simulink model "PS_03_sim"  (R2018a)
settings: Solver=FixedStepDiscrete  StartTime=0.0  StopTime=2376922056.5209  FixedStep=95076882.2608359  RelTol=1e-3
values from neighbouring files (symbols this model uses):
  a = rp/(1-e)    [AA279A_final2019.m]    (also in ECI2OE.m = inf; OEtoRVv2.m = (mu/n^2)^(1/3); PS_03.m = 2667966400; ps_2.m = sqrt( (L^2-2*T*Ix) / ((Iy-Ix)*Iy) ))
  e = 0.2    [AA279A_final2019.m]    (also in ECI2OE.m = norm ( eVec ); PS_03.m = 0.967; plotParabola.m = 1; ps_2.m = sqrt(1 + (b^2/abs(a^2))))
  M0 = 0    [PS_03.m]
  n = 2*pi/T    [AA279A_final2019.m]    (also in ECI2OE.m = norm ( nVec ); OEtoRV.m = sqrt(mu/a^3); PS_03.m = sqrt(mu/a^3); UDFactor.m = length(P))
  tol = 1E-10    (= 1e-10)    [PS_03.m]
settings Model: Creator=kaitl  LastModifiedBy=kaitl

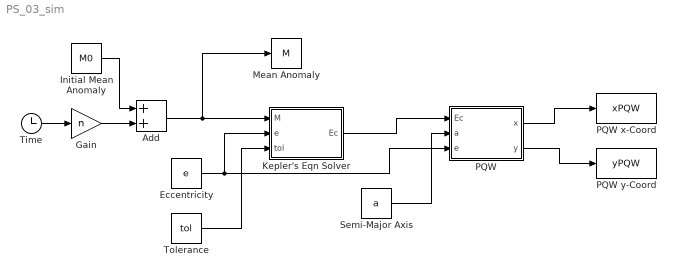
== system PS_03_sim ==
  Add : Sum
  Eccentricity : Constant  Value=e
  Gain : Gain  Gain=n
  Initial Mean Anomaly : Constant  Value=M0
  Kepler's Eqn Solver : MATLAB Function  TreatAsAtomicUnit=on
  Mean Anomaly : ToWorkspace  VariableName=M  SampleTime=-1
  PQW : MATLAB Function  TreatAsAtomicUnit=on
  PQW x-Coord : ToWorkspace  VariableName=xPQW  SampleTime=-1
  PQW y-Coord : ToWorkspace  VariableName=yPQW  SampleTime=-1
  Semi-Major Axis : Constant  Value=a
  Time : Clock
  Tolerance : Constant  Value=tol
  wires:
  Time/1 -> Gain/1
  Gain/1 -> Add/2
  Initial Mean Anomaly/1 -> Add/1
  Add/1 -> Mean Anomaly/1, Kepler's Eqn Solver/1(M)
  Eccentricity/1 -> PQW/3(e), Kepler's Eqn Solver/2(e)
  Tolerance/1 -> Kepler's Eqn Solver/3(tol)
  Kepler's Eqn Solver/1(Ec) -> PQW/1(Ec)
  Semi-Major Axis/1 -> PQW/2(a)
  PQW/1(x) -> PQW x-Coord/1
  PQW/2(y) -> PQW y-Coord/1

== matlab function PS_03_sim/PQW ==
  data: Ec input; x output; a input; y output; e input
function [x,y] = OEtoPQW(Ec,a,e)
x = a*(cos(Ec)-e);
y = a*sqrt(1-e^2)*sin(Ec);
end

== matlab function PS_03_sim/Kepler's Eqn Solver ==
  data: M input; Ec output; e input; tol input
function Ec = MtoEc(M,e,tol)
if M == 0 || M == pi
    Ec = M;
else
    er = 100;
    Ec = M;
    Eco = M;
    iter = 0;
    while er >= tol && iter <= 100
        del = -(Eco-e*sin(Eco)-M)/(1-e*cos(Eco));
        Ec = Eco + del;
        er = abs(Ec-Eco);
        Eco = Ec;
        iter = iter + 1;
    end
end
